simulink model "VehCtrl20260630_18B"  (R2018b)
settings: Solver=FixedStepAuto  StartTime=0.0  StopTime=inf  FixedStep=0.005  RelTol=1e-3
InitFcn:
  | mbd_mpc_consistency_checks(bdroot(gcs));
undefined symbols (not defined in the file): ANG_DEAD, BMS_NormalPwr, BrakeDeadZone, BrkPrsByBrkPct_TB_X, BrkPrsByBrkPct_TB_Y, DELAY_DISCHARGE, DELAY_RCUOFF, DRV_BACKWARD, DRV_BRAKE, DRV_FORWARD, DRV_NEUTRAL, DRV_PARK, DRV_UNPARK, DRV_ZEROTURN, EPB_LOCK, EPB_UNLOCK, ExtraLoadPwr, FanOff, fifo_0_vect, fifo_1_vect, HiFanReq, HV_finished, HV_No_Active, HV_POWER_OFF, HV_POWER_ON, HVDown, HVON, KaTLS_v_DrgUp_X_VehSpd, KeFTM_s_Way1OffDlyTime, KeFTM_TK_Way1CoolLv2OffBatTemp, KeFTM_TK_Way1CoolLv2OffMtrTemp, KeFTM_TK_Way1CoolLv2OnBatTemp, KeFTM_TK_Way1CoolLv2OnMtrTemp, KeFTM_TK_Way1CoolLv3OffBatTemp, KeFTM_TK_Way1CoolLv3OffMtrTemp, KeFTM_TK_Way1CoolLv3OnBatTemp, KeFTM_TK_Way1CoolLv3OnMtrTemp, KeFTM_TK_Way1CoolLv4OffBatTemp, KeFTM_TK_Way1CoolLv4OffMtrTemp, KeFTM_TK_Way1CoolLv4OnBatTemp, KeFTM_TK_Way1CoolLv4OnMtrTemp, Kp1, Kp2, LowFanReq, LQFP, MtrCmdGainFL, MtrCmdGainFR, MtrCmdGainRL, MtrCmdGainRR, MtrPwrFactor_RCU, MtrPwrHighToMidThd, MtrPwrLowToMidThd, MtrPwrMidToHighThd, MtrPwrMidToLowThd, MtrTrqMax, PCT_DEAD, Precharge, PTO_1000, PTO_540, pts1_fifo_0_vect ... (+32)
libraries: mbd_mpc574x_ec_toolbox x175, simulink x110, canmsglib x70
(part 8 of 15)

== system VehCtrl20260630_18B/SigIn/CAN0/DC-DC_Msg/UNPACK ==
  ID : Inport
  data : Inport  Port=2
  length : Inport  Port=3
  timestamp : Inport  Port=4
  Action Port : ActionPort  ActionType=case
  Add : Sum
  Bus Creator : BusCreator  Inputs=7  OutDataTypeStr=Bus: CAN_MESSAGE_BUS  NonVirtualBus=on
  Bus Creator1 : BusCreator  Inputs=8
  CAN Unpack6 : canmsglib/CAN Unpack  CANdbFile=E:\硕士工作\0.本周工作\20260428_changchun\VCU_260508_ChangChun\CAN协议0509\DCDC\DCDC_DBC_VCU_CAN0.dbc  MsgList=DCDC_msg1  MsgName=DCDC_msg1  MsgIDType=Extended (29-bit identifier)  MsgIdentifier=418931243  MsgLength=8  SignalInfo=DCDC_BasicSts$5$3$1$2$1$0$1$0$0$7$#DCDC_ErrorLevel$3$2$1$2$1$0$1$0$0$3$#DCDC_FaultLevel$48$8$1$2$1$0$1$0$0$200$#DCDC_Mdltem$8$8$1$2$1$0$1$-40$-40$150$#DCDC_Optcur$32$16$1$2$1$0$5.000000e-02$0$0$3.276750e+03$#DCDC_Optvol$16$16$1$2$1$0$5.000000e-02$0$0$3.276750e+03$#DCDC_Sfwver$56$8$1$2$1$0$1$0$1$255$#DCDC_WrkSts$1$2$1$2$1$0$1$0$0$3$#Spare$0$1$1$2$1$0$1$0$0$1$#  NSignals=9  IDPort=off  TimestampPort=off  ErrorPort=off  RemotePort=off  LengthPort=off  StatusPort=off  StartBits=str2num('[int32(5);int32(3);int32(48);int32(8);int32(32);int32(16);int32(56);int32(1);int32(0)]')  SignalSizes=str2num('[int32(3);int32(2);int32(8);int32(8);int32(16);int32(16);int32(8);int32(2);int32(1)]')  ByteOrders=str2num('[int32(1);int32(1);int32(1);int32(1);int32(1);int32(1);int32(1);int32(1);int32(1)]')  DataTypes=str2num('[int32(2);int32(2);int32(2);int32(2);int32(2);int32(2);int32(2);int32(2);int32(2)]')  MultiplexTypes=str2num('[int32(1);int32(1);int32(1);int32(1);int32(1);int32(1);int32(1);int32(1);int32(1)]')  MultiplexValues=str2num('[double(0);double(0);double(0);double(0);double(0);double(0);double(0);double(0);double(0)]')  Factors=str2num('[double(1);double(1);double(1);double(1);double(5.000000e-02);double(5.000000e-02);double(1);double(1);double(1)]')  Offsets=str2num('[double(0);double(0);double(0);double(-40);double(0);double(0);double(0);double(0);double(0)]')  Minimums=str2num('[double(0);double(0);double(0);double(-40);double(0);double(0);double(1);double(0);double(0)]')  Maximums=str2num('[double(7);double(3);double(200);double(150);double(3.276750e+03);double(3.276750e+03);double(255);double(3);double(1)]')  ApplyMinMax=off
      settings: SourceProductName=Simulink Real-Time  SourceProductBaseCode=XP  DataFormat=CANdb specified signals
  Constant : Constant  OutDataTypeStr=uint8
  Constant1 : Constant  OutDataTypeStr=uint8
  Constant4 : Constant  Value=0  OutDataTypeStr=uint8
  Constant5 : Constant  Value=0  OutDataTypeStr=uint8
  Data Store Read : DataStoreRead  DataStoreName=Cnt_DCDC
  Data Store Write : DataStoreWrite  DataStoreName=Cnt_DCDC
  Data Type Conversion{,14..15,17} (4 alike) : DataTypeConversion  OutDataTypeStr=uint8
  Data Type Conversion{1..6,61..62} (8 alike) : DataTypeConversion  OutDataTypeStr=single
  Data Type Conversion18 : DataTypeConversion  OutDataTypeStr=uint32
  Data Type Conversion19 : DataTypeConversion  OutDataTypeStr=double
  Terminator : Terminator
  Message : Outport
  wires:
  Constant4/1 -> Data Type Conversion15/1
  length/1 -> Data Type Conversion14/1
  data/1 -> Bus Creator/7  "Data"
  Data Type Conversion18/1 -> Bus Creator/5  "ID"
  Constant1/1 -> Data Type Conversion/1
  Constant5/1 -> Data Type Conversion17/1
  ID/1 -> Data Type Conversion18/1
  Data Type Conversion19/1 -> Bus Creator/6  "Timestamp"
  timestamp/1 -> Data Type Conversion19/1
  Data Type Conversion17/1 -> Bus Creator/4  "Error"
  Bus Creator/1 -> CAN Unpack6/1  "CAN_Msg_In"
  Data Type Conversion/1 -> Bus Creator/1  "Extended"
  Data Type Conversion14/1 -> Bus Creator/2  "Length"
  Data Type Conversion15/1 -> Bus Creator/3  "Remote"
  Bus Creator1/1 -> Message/1
  Data Type Conversion4/1 -> Bus Creator1/1  "DCDC_BasicSts"
  Data Type Conversion61/1 -> Bus Creator1/2  "DCDC_ErrorLevel"
  Data Type Conversion62/1 -> Bus Creator1/3  "DCDC_FaultLevel"
  Data Type Conversion2/1 -> Bus Creator1/4  "DCDC_Mdltem"
  Data Type Conversion1/1 -> Bus Creator1/5  "DCDC_Optcur"
  CAN Unpack6/9 -> Terminator/1
  Data Type Conversion3/1 -> Bus Creator1/6  "DCDC_Optvol"
  Data Type Conversion5/1 -> Bus Creator1/7  "DCDC_Sfwver"
  Data Type Conversion6/1 -> Bus Creator1/8  "DCDC_WrkSts"
  CAN Unpack6/1 -> Data Type Conversion4/1
  CAN Unpack6/2 -> Data Type Conversion61/1
  CAN Unpack6/3 -> Data Type Conversion62/1
  CAN Unpack6/4 -> Data Type Conversion2/1
  CAN Unpack6/5 -> Data Type Conversion1/1
  CAN Unpack6/6 -> Data Type Conversion3/1
  CAN Unpack6/7 -> Data Type Conversion5/1
  CAN Unpack6/8 -> Data Type Conversion6/1
  Add/1 -> Data Store Write/1
  Constant/1 -> Add/2
  Data Store Read/1 -> Add/1

== system VehCtrl20260630_18B/SigIn/CAN0/PTC1/UNPACK ==
  ID : Inport
  data : Inport  Port=2
  length : Inport  Port=3
  timestamp : Inport  Port=4
  Action Port : ActionPort  ActionType=case
  Bus Creator : BusCreator  Inputs=7  OutDataTypeStr=Bus: CAN_MESSAGE_BUS  NonVirtualBus=on
  Bus Creator1 : BusCreator  Inputs=7
  CAN Unpack6 : canmsglib/CAN Unpack  CANdbFile=D:\VCU\VCU_AgriculturalMachinery_ChangChun\CAN协议8.4\PTC\PTC_Sheet1.dbc  MsgList=PTC_1  MsgName=PTC_1  MsgIDType=Standard (11-bit identifier)  MsgIdentifier=1179  MsgLength=8  SignalInfo=PTC_Actualdutycycle$56$8$2$2$1$0$1$0$0$100$#PTC_Consumedpower$24$16$2$2$1$0$2$0$0$16000$#PTC_Coolanttemperature$48$8$2$2$1$0$1$-40$0$140$#PTC_IGBTheatsinktemperature$40$8$2$2$1$0$1$-40$0$140$#PTC_Operatingcurrent$0$8$2$2$1$0$2.000000e-01$0$0$50$#PTC_Workingcurrent$8$8$2$2$1$0$2.000000e-01$0$0$50$#PTC_Workingvoltage$16$8$2$2$1$0$4$0$0$1000$#  NSignals=7  IDPort=off  TimestampPort=off  ErrorPort=off  RemotePort=off  LengthPort=off  StatusPort=off  StartBits=str2num('[int32(56);int32(24);int32(48);int32(40);int32(0);int32(8);int32(16)]')  SignalSizes=str2num('[int32(8);int32(16);int32(8);int32(8);int32(8);int32(8);int32(8)]')  ByteOrders=str2num('[int32(2);int32(2);int32(2);int32(2);int32(2);int32(2);int32(2)]')  DataTypes=str2num('[int32(2);int32(2);int32(2);int32(2);int32(2);int32(2);int32(2)]')  MultiplexTypes=str2num('[int32(1);int32(1);int32(1);int32(1);int32(1);int32(1);int32(1)]')  MultiplexValues=str2num('[double(0);double(0);double(0);double(0);double(0);double(0);double(0)]')  Factors=str2num('[double(1);double(2);double(1);double(1);double(2.000000e-01);double(2.000000e-01);double(4)]')  Offsets=str2num('[double(0);double(0);double(-40);double(-40);double(0);double(0);double(0)]')  Minimums=str2num('[double(0);double(0);double(0);double(0);double(0);double(0);double(0)]')  Maximums=str2num('[double(100);double(16000);double(140);double(140);double(50);double(50);double(1000)]')  ApplyMinMax=off
      settings: SourceProductName=Simulink Real-Time  SourceProductBaseCode=XP  DataFormat=CANdb specified signals
  Constant1 : Constant  OutDataTypeStr=uint8
  Constant4 : Constant  Value=0  OutDataTypeStr=uint8
  Constant5 : Constant  Value=0  OutDataTypeStr=uint8
  Data Type Conversion{,14..15,17} (4 alike) : DataTypeConversion  OutDataTypeStr=uint8
  Data Type Conversion{1..5,61..62} (7 alike) : DataTypeConversion  OutDataTypeStr=single
  Data Type Conversion18 : DataTypeConversion  OutDataTypeStr=uint32
  Data Type Conversion19 : DataTypeConversion  OutDataTypeStr=double
  Message : Outport
  wires:
  Constant4/1 -> Data Type Conversion15/1
  length/1 -> Data Type Conversion14/1
  data/1 -> Bus Creator/7  "Data"
  Data Type Conversion18/1 -> Bus Creator/5  "ID"
  Constant1/1 -> Data Type Conversion/1
  Constant5/1 -> Data Type Conversion17/1
  ID/1 -> Data Type Conversion18/1
  Data Type Conversion19/1 -> Bus Creator/6  "Timestamp"
  timestamp/1 -> Data Type Conversion19/1
  Data Type Conversion17/1 -> Bus Creator/4  "Error"
  Bus Creator/1 -> CAN Unpack6/1  "CAN_Msg_In"
  Data Type Conversion/1 -> Bus Creator/1  "Extended"
  Data Type Conversion14/1 -> Bus Creator/2  "Length"
  Data Type Conversion15/1 -> Bus Creator/3  "Remote"
  Bus Creator1/1 -> Message/1
  Data Type Conversion4/1 -> Bus Creator1/1  "PTC_Actualdutycycle"
  Data Type Conversion61/1 -> Bus Creator1/2  "PTC_Consumedpower"
  Data Type Conversion62/1 -> Bus Creator1/3  "PTC_Coolanttemperature"
  Data Type Conversion2/1 -> Bus Creator1/4  "PTC_IGBTheatsinktemperature"
  Data Type Conversion1/1 -> Bus Creator1/5  "PTC_Operatingcurrent"
  Data Type Conversion3/1 -> Bus Creator1/6  "PTC_Workingcurrent"
  Data Type Conversion5/1 -> Bus Creator1/7  "PTC_Workingvoltage"
  CAN Unpack6/1 -> Data Type Conversion4/1
  CAN Unpack6/2 -> Data Type Conversion61/1
  CAN Unpack6/3 -> Data Type Conversion62/1
  CAN Unpack6/4 -> Data Type Conversion2/1
  CAN Unpack6/5 -> Data Type Conversion1/1
  CAN Unpack6/6 -> Data Type Conversion3/1
  CAN Unpack6/7 -> Data Type Conversion5/1

== system VehCtrl20260630_18B/SigIn/CAN0/PTC2/UNPACK ==
  ID : Inport
  data : Inport  Port=2
  length : Inport  Port=3
  timestamp : Inport  Port=4
  Action Port : ActionPort  ActionType=case
  Bus Creator : BusCreator  Inputs=7  OutDataTypeStr=Bus: CAN_MESSAGE_BUS  NonVirtualBus=on
  Bus Creator1 : BusCreator  Inputs=11
  CAN Unpack6 : canmsglib/CAN Unpack  CANdbFile=D:\VCU\VCU_AgriculturalMachinery_ChangChun\CAN协议8.4\PTC\PTC_Sheet1.dbc  MsgList=PTC_2  MsgName=PTC_2  MsgIDType=Standard (11-bit identifier)  MsgIdentifier=1180  MsgLength=4  SignalInfo=PTC_Highvoltagecircuitdisconnection$6$2$2$2$1$0$1$0$0$3$#PTC_Highvoltagepowersupplycondition$4$2$2$2$1$0$1$0$0$3$#PTC_IG1powersupplyisfaulty$14$2$2$2$1$0$1$0$0$3$#PTC_IGBTshortcircuit$18$1$2$2$1$0$1$0$0$1$#PTC_Numberofsoftwaremodifications$24$8$2$2$1$0$1$0$0$255$#PTC_Requesttodisconnecttheairconditionercontactor$16$2$2$2$1$0$1$0$0$3$#PTC_coolanttemperaturesensorisfaulty$12$2$2$2$1$0$1$0$0$3$#PTC_enabledSts$0$2$2$2$1$0$1$0$0$3$#PTC_faultySts$2$2$2$2$1$0$1$0$0$3$#TheIGBTtemperaturesensorisfaulty$10$2$2$2$1$0$1$0$0$3$#Thecommunicationwiththeairconditionercontrollerislost$8$2$2$2$1$0$1$0$0$3$#  NSignals=11  IDPort=off  TimestampPort=off  ErrorPort=off  RemotePort=off  LengthPort=off  StatusPort=off  StartBits=str2num('[int32(6);int32(4);int32(14);int32(18);int32(24);int32(16);int32(12);int32(0);int32(2);int32(10);int32(8)]')  SignalSizes=str2num('[int32(2);int32(2);int32(2);int32(1);int32(8);int32(2);int32(2);int32(2);int32(2);int32(2);int32(2)]')  ByteOrders=str2num('[int32(2);int32(2);int32(2);int32(2);int32(2);int32(2);int32(2);int32(2);int32(2);int32(2);int32(2)]')  DataTypes=str2num('[int32(2);int32(2);int32(2);int32(2);int32(2);int32(2);int32(2);int32(2);int32(2);int32(2);int32(2)]')  MultiplexTypes=str2num('[int32(1);int32(1);int32(1);int32(1);int32(1);int32(1);int32(1);int32(1);int32(1);int32(1);int32(1)]')  MultiplexValues=str2num('[double(0);double(0);double(0);double(0);double(0);double(0);double(0);double(0);double(0);double(0);double(0)]')  Factors=str2num('[double(1);double(1);double(1);double(1);double(1);double(1);double(1);double(1);double(1);double(1);double(1)]')  Offsets=str2num('[double(0);double(0);double(0);double(0);double(0);double(0);double(0);double(0);double(0);double(0);double(0)]')  Minimums=str2num('[double(0);double(0);double(0);double(0);double(0);double(0);double(0);double(0);double(0);double(0);double(0)]')  Maximums=str2num('[double(3);double(3);double(3);double(1);double(255);double(3);double(3);double(3);double(3);double(3);double(3)]')  ApplyMinMax=off
      settings: SourceProductName=Simulink Real-Time  SourceProductBaseCode=XP  DataFormat=CANdb specified signals
  Constant1 : Constant  OutDataTypeStr=uint8
  Constant4 : Constant  Value=0  OutDataTypeStr=uint8
  Constant5 : Constant  Value=0  OutDataTypeStr=uint8
  Data Type Conversion{,2..9,14..15,17,61..62} (14 alike) : DataTypeConversion  OutDataTypeStr=uint8
  Data Type Conversion1 : DataTypeConversion  OutDataTypeStr=single
  Data Type Conversion18 : DataTypeConversion  OutDataTypeStr=uint32
  Data Type Conversion19 : DataTypeConversion  OutDataTypeStr=double
  Message : Outport
  wires:
  Constant4/1 -> Data Type Conversion15/1
  length/1 -> Data Type Conversion14/1
  data/1 -> Bus Creator/7  "Data"
  Data Type Conversion18/1 -> Bus Creator/5  "ID"
  Constant1/1 -> Data Type Conversion/1
  Constant5/1 -> Data Type Conversion17/1
  ID/1 -> Data Type Conversion18/1
  Data Type Conversion19/1 -> Bus Creator/6  "Timestamp"
  timestamp/1 -> Data Type Conversion19/1
  Data Type Conversion17/1 -> Bus Creator/4  "Error"
  Bus Creator/1 -> CAN Unpack6/1  "CAN_Msg_In"
  Data Type Conversion/1 -> Bus Creator/1  "Extended"
  Data Type Conversion14/1 -> Bus Creator/2  "Length"
  Data Type Conversion15/1 -> Bus Creator/3  "Remote"
  Bus Creator1/1 -> Message/1
  Data Type Conversion4/1 -> Bus Creator1/1  "PTC_Highvoltagepowersupplycondition"
  Data Type Conversion61/1 -> Bus Creator1/2  "PTC_Highvoltagecircuitdisconnection"
  Data Type Conversion62/1 -> Bus Creator1/3  "PTC_IG1powersupplyisfaulty"
  Data Type Conversion2/1 -> Bus Creator1/4  "PTC_IGBTshortcircuit"
  Data Type Conversion1/1 -> Bus Creator1/5  "PTC_Numberofsoftwaremodifications"
  CAN Unpack6/9 -> Data Type Conversion7/1
  Data Type Conversion3/1 -> Bus Creator1/6  "PTC_Requesttodisconnecttheairconditionercontactor"
  Data Type Conversion5/1 -> Bus Creator1/7  "PTC_coolanttemperaturesensorisfaulty"
  Data Type Conversion6/1 -> Bus Creator1/8  "PTC_enabledSts"
  CAN Unpack6/1 -> Data Type Conversion4/1
  CAN Unpack6/2 -> Data Type Conversion61/1
  CAN Unpack6/3 -> Data Type Conversion62/1
  CAN Unpack6/4 -> Data Type Conversion2/1
  CAN Unpack6/5 -> Data Type Conversion1/1
  CAN Unpack6/6 -> Data Type Conversion3/1
  CAN Unpack6/7 -> Data Type Conversion5/1
  CAN Unpack6/8 -> Data Type Conversion6/1
  Data Type Conversion7/1 -> Bus Creator1/9  "PTC_faulty Sts"
  Data Type Conversion8/1 -> Bus Creator1/10  "TheIGBTtemperaturesensorisfaulty"
  CAN Unpack6/10 -> Data Type Conversion8/1
  Data Type Conversion9/1 -> Bus Creator1/11  "Thecommunicationwiththeairconditionercontrollerislost"
  CAN Unpack6/11 -> Data Type Conversion9/1

== system VehCtrl20260630_18B/SigIn/CAN0/RMT_VCU1/UNPACK ==
  ID : Inport
  data : Inport  Port=2
  length : Inport  Port=3
  timestamp : Inport  Port=4
  Action Port : ActionPort  ActionType=case
  Add : Sum
  Bus Creator : BusCreator  Inputs=7  OutDataTypeStr=Bus: CAN_MESSAGE_BUS  NonVirtualBus=on
  Bus Creator1 : BusCreator  Inputs=3
  CAN Unpack6 : canmsglib/CAN Unpack  CANdbFile=E:\硕士工作\0.本周工作\20260428_changchun\VCU_260508_ChangChun\CAN协议0430\RMT\CAN_Matrix_Sheet1_0509.dbc  MsgList=JoyStick  MsgName=JoyStick  MsgIDType=Standard (11-bit identifier)  MsgIdentifier=1  MsgLength=8  SignalInfo=CmdAccBrkPct$32$16$1$2$1$0$1$0$0$100$#CmdSteerAng$0$16$1$2$1$0$1$0$0$100$#ReserveL$48$16$1$2$1$0$1$0$0$100$#ReserveR$16$16$1$2$1$0$1$0$0$100$#  NSignals=4  IDPort=off  TimestampPort=off  ErrorPort=off  RemotePort=off  LengthPort=off  StatusPort=off  StartBits=str2num('[int32(32);int32(0);int32(48);int32(16)]')  SignalSizes=str2num('[int32(16);int32(16);int32(16);int32(16)]')  ByteOrders=str2num('[int32(1);int32(1);int32(1);int32(1)]')  DataTypes=str2num('[int32(2);int32(2);int32(2);int32(2)]')  MultiplexTypes=str2num('[int32(1);int32(1);int32(1);int32(1)]')  MultiplexValues=str2num('[double(0);double(0);double(0);double(0)]')  Factors=str2num('[double(1);double(1);double(1);double(1)]')  Offsets=str2num('[double(0);double(0);double(0);double(0)]')  Minimums=str2num('[double(0);double(0);double(0);double(0)]')  Maximums=str2num('[double(100);double(100);double(100);double(100)]')  ApplyMinMax=off
      settings: SourceProductName=Simulink Real-Time  SourceProductBaseCode=XP  DataFormat=CANdb specified signals
  Constant : Constant  OutDataTypeStr=uint8
  Constant1 : Constant  Value=0  OutDataTypeStr=uint8
  Constant4 : Constant  Value=0  OutDataTypeStr=uint8
  Constant5 : Constant  Value=0  OutDataTypeStr=uint8
  Data Store Read : DataStoreRead  DataStoreName=Cnt_RMT1
  Data Store Write : DataStoreWrite  DataStoreName=Cnt_RMT1
  Data Type Conversion{,14..15,17} (4 alike) : DataTypeConversion  OutDataTypeStr=uint8
  Data Type Conversion1 : DataTypeConversion  OutDataTypeStr=single
  Data Type Conversion18 : DataTypeConversion  OutDataTypeStr=uint32
  Data Type Conversion19 : DataTypeConversion  OutDataTypeStr=double
  Data Type Conversion61 : DataTypeConversion  OutDataTypeStr=single
  Subsystem : Subsystem
  Subsystem1 : Subsystem
  Subsystem2 : Subsystem
  Terminator : Terminator
  Terminator1 : Terminator
  Message : Outport
  wires:
  Constant4/1 -> Data Type Conversion15/1
  length/1 -> Data Type Conversion14/1
  data/1 -> Bus Creator/7  "Data"
  Data Type Conversion18/1 -> Bus Creator/5  "ID"
  Constant1/1 -> Data Type Conversion/1
  Constant5/1 -> Data Type Conversion17/1
  ID/1 -> Data Type Conversion18/1
  Data Type Conversion19/1 -> Bus Creator/6  "Timestamp"
  timestamp/1 -> Data Type Conversion19/1
  Data Type Conversion17/1 -> Bus Creator/4  "Error"
  Bus Creator/1 -> CAN Unpack6/1  "CAN_Msg_In"
  Data Type Conversion/1 -> Bus Creator/1  "Extended"
  Data Type Conversion14/1 -> Bus Creator/2  "Length"
  Data Type Conversion15/1 -> Bus Creator/3  "Remote"
  Bus Creator1/1 -> Message/1
  Data Type Conversion61/1 -> Subsystem1/1(In1), Subsystem/1(In1)  "RMT_CmdAccBrkSig"
  Subsystem2/1(Out1) -> Bus Creator1/3  "RMT_CmdStrAng"
  CAN Unpack6/1 -> Data Type Conversion61/1
  Add/1 -> Data Store Write/1
  Constant/1 -> Add/2
  Data Store Read/1 -> Add/1
  Subsystem/1(Out1) -> Bus Creator1/1  "RMT_CmdAccPct"
  Subsystem1/1(Out1) -> Bus Creator1/2  "RMT_CmdBrkPct"
  CAN Unpack6/2 -> Data Type Conversion1/1
  Data Type Conversion1/1 -> Subsystem2/1(In1)  "RMT_CmdStrSig"
  CAN Unpack6/3 -> Terminator/1
  CAN Unpack6/4 -> Terminator1/1

== system VehCtrl20260630_18B/SigIn/CAN0/RMT_VCU2/UNPACK ==
  ID : Inport
  data : Inport  Port=2
  length : Inport  Port=3
  timestamp : Inport  Port=4
  Action Port : ActionPort  ActionType=case
  Add : Sum
  Bus Creator : BusCreator  Inputs=7  OutDataTypeStr=Bus: CAN_MESSAGE_BUS  NonVirtualBus=on
  Bus Creator1 : BusCreator  Inputs=3
  CAN Unpack6 : canmsglib/CAN Unpack  CANdbFile=E:\硕士工作\0.本周工作\20260428_changchun\VCU_260508_ChangChun\CAN协议0430\RMT\CAN_Matrix_Sheet1_0509.dbc  MsgList=VR  MsgName=VR  MsgIDType=Standard (11-bit identifier)  MsgIdentifier=2  MsgLength=8  SignalInfo=CmdLiftPct$32$16$1$2$1$0$1$0$0$100$#CmdTrackWidthPct$0$16$1$2$1$0$1$0$0$100$#MotorTorqueGear$16$16$1$2$1$0$1$0$0$100$#ReserveVRB$48$16$1$2$1$0$1$0$0$100$#  NSignals=4  IDPort=off  TimestampPort=off  ErrorPort=off  RemotePort=off  LengthPort=off  StatusPort=off  StartBits=str2num('[int32(32);int32(0);int32(16);int32(48)]')  SignalSizes=str2num('[int32(16);int32(16);int32(16);int32(16)]')  ByteOrders=str2num('[int32(1);int32(1);int32(1);int32(1)]')  DataTypes=str2num('[int32(2);int32(2);int32(2);int32(2)]')  MultiplexTypes=str2num('[int32(1);int32(1);int32(1);int32(1)]')  MultiplexValues=str2num('[double(0);double(0);double(0);double(0)]')  Factors=str2num('[double(1);double(1);double(1);double(1)]')  Offsets=str2num('[double(0);double(0);double(0);double(0)]')  Minimums=str2num('[double(0);double(0);double(0);double(0)]')  Maximums=str2num('[double(100);double(100);double(100);double(100)]')  ApplyMinMax=off
      settings: SourceProductName=Simulink Real-Time  SourceProductBaseCode=XP  DataFormat=CANdb specified signals
  Constant : Constant  OutDataTypeStr=uint8
  Constant1 : Constant  Value=0  OutDataTypeStr=uint8
  Constant4 : Constant  Value=0  OutDataTypeStr=uint8
  Constant5 : Constant  Value=0  OutDataTypeStr=uint8
  Data Store Read : DataStoreRead  DataStoreName=Cnt_RMT2
  Data Store Write : DataStoreWrite  DataStoreName=Cnt_RMT2
  Data Store Write1 : DataStoreWrite  Commented=on  DataStoreName=MtrTrqGr
  Data Type Conversion{,14..15,17} (4 alike) : DataTypeConversion  OutDataTypeStr=uint8
  Data Type Conversion1 : DataTypeConversion  OutDataTypeStr=single
  Data Type Conversion18 : DataTypeConversion  OutDataTypeStr=uint32
  Data Type Conversion19 : DataTypeConversion  OutDataTypeStr=double
  Data Type Conversion2 : DataTypeConversion  OutDataTypeStr=single
  Data Type Conversion3 : DataTypeConversion  OutDataTypeStr=single
  Subsystem : Subsystem
  Subsystem3 : Subsystem
  Subsystem4 : Subsystem
  Terminator : Terminator
  Message : Outport
  wires:
  Bus Creator1/1 -> Message/1
  Data Type Conversion15/1 -> Bus Creator/3  "Remote"
  Data Type Conversion14/1 -> Bus Creator/2  "Length"
  Data Type Conversion/1 -> Bus Creator/1  "Extended"
  Bus Creator/1 -> CAN Unpack6/1  "CAN_Msg_In"
  Data Type Conversion17/1 -> Bus Creator/4  "Error"
  timestamp/1 -> Data Type Conversion19/1
  Data Type Conversion19/1 -> Bus Creator/6  "Timestamp"
  ID/1 -> Data Type Conversion18/1
  Constant5/1 -> Data Type Conversion17/1
  Constant1/1 -> Data Type Conversion/1
  Data Type Conversion18/1 -> Bus Creator/5  "ID"
  data/1 -> Bus Creator/7  "Data"
  length/1 -> Data Type Conversion14/1
  Constant4/1 -> Data Type Conversion15/1
  Add/1 -> Data Store Write/1
  Constant/1 -> Add/2
  Data Store Read/1 -> Add/1
  Data Type Conversion1/1 -> Subsystem/1(RMT_MtrTqGr)
  Subsystem/1(Out1) -> Data Store Write1/1, Bus Creator1/3  "RMT_MtrTqGr"
  CAN Unpack6/4 -> Terminator/1
  CAN Unpack6/3 -> Data Type Conversion1/1
  Data Type Conversion3/1 -> Subsystem3/1(In1)  "RMT_CmdLiftSig"
  Subsystem3/1(Out1) -> Bus Creator1/1  "RMT_ModeSusp"
  CAN Unpack6/1 -> Data Type Conversion3/1
  Subsystem4/1(Out1) -> Bus Creator1/2  "RMT_ModeWidth"
  Data Type Conversion2/1 -> Subsystem4/1(In1)  "RMT_CmdWidthSig"
  CAN Unpack6/2 -> Data Type Conversion2/1

== system VehCtrl20260630_18B/SigIn/CAN0/RMT_VCU3/UNPACK ==
  note: 1 - 自动驾驶
      | 0 - 遥控
  note: 1 - 急停
      | 0 - 无效
  ID : Inport
  data : Inport  Port=2
  length : Inport  Port=3
  timestamp : Inport  Port=4
  Action Port : ActionPort  ActionType=case
  Add : Sum
  Bus Creator : BusCreator  Inputs=7  OutDataTypeStr=Bus: CAN_MESSAGE_BUS  NonVirtualBus=on
  Bus Creator1 : BusCreator  Inputs=4
  CAN Unpack6 : canmsglib/CAN Unpack  CANdbFile=D:\VCU\VCU_AgriculturalMachinery_ChangChun\VCU_AgriculturalMachinery_260520_ChangChun\CAN协议0520\RMT\RMT_dbc1.dbc  MsgList=SW1  MsgName=SW1  MsgIDType=Standard (11-bit identifier)  MsgIdentifier=3  MsgLength=8  SignalInfo=CoachSwitch$48$16$1$2$1$0$1$0$0$100$#EmStop$16$16$1$2$1$0$1$0$0$100$#ModeDirection$0$16$1$2$1$0$1$0$0$100$#ReserveH$32$16$1$2$1$0$1$0$0$100$#  NSignals=4  IDPort=off  TimestampPort=off  ErrorPort=off  RemotePort=off  LengthPort=off  StatusPort=off  StartBits=str2num('[int32(48);int32(16);int32(0);int32(32)]')  SignalSizes=str2num('[int32(16);int32(16);int32(16);int32(16)]')  ByteOrders=str2num('[int32(1);int32(1);int32(1);int32(1)]')  DataTypes=str2num('[int32(2);int32(2);int32(2);int32(2)]')  MultiplexTypes=str2num('[int32(1);int32(1);int32(1);int32(1)]')  MultiplexValues=str2num('[double(0);double(0);double(0);double(0)]')  Factors=str2num('[double(1);double(1);double(1);double(1)]')  Offsets=str2num('[double(0);double(0);double(0);double(0)]')  Minimums=str2num('[double(0);double(0);double(0);double(0)]')  Maximums=str2num('[double(100);double(100);double(100);double(100)]')  ApplyMinMax=off
      settings: SourceProductName=Simulink Real-Time  SourceProductBaseCode=XP  DataFormat=CANdb specified signals
  Constant : Constant  OutDataTypeStr=uint8
  Constant1 : Constant  Value=0  OutDataTypeStr=uint8
  Constant4 : Constant  Value=0  OutDataTypeStr=uint8
  Constant5 : Constant  Value=0  OutDataTypeStr=uint8
  Data Store Read : DataStoreRead  DataStoreName=Cnt_RMT3
  Data Store Write : DataStoreWrite  DataStoreName=Cnt_RMT3
  Data Store Write1 : DataStoreWrite  DataStoreName=EmStop_RMT
  Data Type Conversion{,14..15,17} (4 alike) : DataTypeConversion  OutDataTypeStr=uint8
  Data Type Conversion{1,3,6..7} (4 alike) : DataTypeConversion  OutDataTypeStr=single
  Data Type Conversion18 : DataTypeConversion  OutDataTypeStr=uint32
  Data Type Conversion19 : DataTypeConversion  OutDataTypeStr=double
  Subsystem1 : Subsystem
  Subsystem2 : Subsystem
  Subsystem4 : Subsystem
  Subsystem5 : Subsystem
  Message : Outport
  wires:
  Constant4/1 -> Data Type Conversion15/1
  length/1 -> Data Type Conversion14/1
  data/1 -> Bus Creator/7  "Data"
  Data Type Conversion18/1 -> Bus Creator/5  "ID"
  Constant1/1 -> Data Type Conversion/1
  Constant5/1 -> Data Type Conversion17/1
  ID/1 -> Data Type Conversion18/1
  Data Type Conversion19/1 -> Bus Creator/6  "Timestamp"
  timestamp/1 -> Data Type Conversion19/1
  Data Type Conversion17/1 -> Bus Creator/4  "Error"
  Bus Creator/1 -> CAN Unpack6/1  "CAN_Msg_In"
  Data Type Conversion/1 -> Bus Creator/1  "Extended"
  Data Type Conversion14/1 -> Bus Creator/2  "Length"
  Data Type Conversion15/1 -> Bus Creator/3  "Remote"
  Add/1 -> Data Store Write/1
  Constant/1 -> Add/2
  Data Store Read/1 -> Add/1
  Data Type Conversion3/1 -> Subsystem1/1(In1)  "RMT_G"
  Bus Creator1/1 -> Message/1
  Data Type Conversion6/1 -> Subsystem4/1(In1)  "RMT_B"
  Data Type Conversion7/1 -> Subsystem5/1(In1)  "RMT_A"
  Subsystem2/1(Out1) -> Bus Creator1/1  "RMT_Auto"
  CAN Unpack6/1 -> Data Type Conversion1/1
  Data Type Conversion1/1 -> Subsystem2/1(In1)  "RMT_H"
  CAN Unpack6/3 -> Data Type Conversion6/1
  Subsystem4/1(Out1) -> Bus Creator1/3  "RMT_ModeDirection"
  Subsystem5/1(Out1) -> Data Store Write1/1, Bus Creator1/2  "RMT_EmStop"
  Subsystem1/1(Out1) -> Bus Creator1/4  "ReserveH"
  CAN Unpack6/4 -> Data Type Conversion3/1
  CAN Unpack6/2 -> Data Type Conversion7/1

== system VehCtrl20260630_18B/SigIn/CAN0/RMT_VCU4/UNPACK ==
  ID : Inport
  data : Inport  Port=2
  length : Inport  Port=3
  timestamp : Inport  Port=4
  Action Port : ActionPort  ActionType=case
  Add : Sum
  Bus Creator : BusCreator  Inputs=7  OutDataTypeStr=Bus: CAN_MESSAGE_BUS  NonVirtualBus=on
  Bus Creator1 : BusCreator  Inputs=3
  CAN Unpack6 : canmsglib/CAN Unpack  CANdbFile=D:\VCU\VCU_AgriculturalMachinery_ChangChun\VCU_AgriculturalMachinery_260520_ChangChun\CAN协议0520\RMT\RMT_dbc1.dbc  MsgList=SW2  MsgName=SW2  MsgIDType=Standard (11-bit identifier)  MsgIdentifier=4  MsgLength=8  SignalInfo=ModeSafety$0$16$1$2$1$0$1$0$0$100$#PowerSwitch$32$16$1$2$1$0$1$0$0$100$#PtoMode$16$16$1$2$1$0$1$0$0$100$#RangeExtenderMode$48$16$1$2$1$0$1$0$0$100$#  NSignals=4  IDPort=off  TimestampPort=off  ErrorPort=off  RemotePort=off  LengthPort=off  StatusPort=off  StartBits=str2num('[int32(0);int32(32);int32(16);int32(48)]')  SignalSizes=str2num('[int32(16);int32(16);int32(16);int32(16)]')  ByteOrders=str2num('[int32(1);int32(1);int32(1);int32(1)]')  DataTypes=str2num('[int32(2);int32(2);int32(2);int32(2)]')  MultiplexTypes=str2num('[int32(1);int32(1);int32(1);int32(1)]')  MultiplexValues=str2num('[double(0);double(0);double(0);double(0)]')  Factors=str2num('[double(1);double(1);double(1);double(1)]')  Offsets=str2num('[double(0);double(0);double(0);double(0)]')  Minimums=str2num('[double(0);double(0);double(0);double(0)]')  Maximums=str2num('[double(100);double(100);double(100);double(100)]')  ApplyMinMax=off
      settings: SourceProductName=Simulink Real-Time  SourceProductBaseCode=XP  DataFormat=CANdb specified signals
  Constant : Constant  OutDataTypeStr=uint8
  Constant1 : Constant  Value=0  OutDataTypeStr=uint8
  Constant4 : Constant  Value=0  OutDataTypeStr=uint8
  Constant5 : Constant  Value=0  OutDataTypeStr=uint8
  Data Store Read : DataStoreRead  DataStoreName=Cnt_RMT4
  Data Store Write : DataStoreWrite  DataStoreName=Cnt_RMT4
  Data Store Write1 : DataStoreWrite  DataStoreName=KeySW
  Data Type Conversion{,14..15,17} (4 alike) : DataTypeConversion  OutDataTypeStr=uint8
  Data Type Conversion{1,3..5} (4 alike) : DataTypeConversion  OutDataTypeStr=single
  Data Type Conversion18 : DataTypeConversion  OutDataTypeStr=uint32
  Data Type Conversion19 : DataTypeConversion  OutDataTypeStr=double
  Data Type Conversion2 : DataTypeConversion
  Subsystem1 : Subsystem
  Subsystem2 : Subsystem
  Subsystem3 : Subsystem
  Subsystem4 : Subsystem
  Message : Outport
  wires:
  Constant4/1 -> Data Type Conversion15/1
  length/1 -> Data Type Conversion14/1
  data/1 -> Bus Creator/7  "Data"
  Data Type Conversion18/1 -> Bus Creator/5  "ID"
  Constant1/1 -> Data Type Conversion/1
  Constant5/1 -> Data Type Conversion17/1
  ID/1 -> Data Type Conversion18/1
  Data Type Conversion19/1 -> Bus Creator/6  "Timestamp"
  timestamp/1 -> Data Type Conversion19/1
  Data Type Conversion17/1 -> Bus Creator/4  "Error"
  Bus Creator/1 -> CAN Unpack6/1  "CAN_Msg_In"
  Data Type Conversion/1 -> Bus Creator/1  "Extended"
  Data Type Conversion14/1 -> Bus Creator/2  "Length"
  Data Type Conversion15/1 -> Bus Creator/3  "Remote"
  Bus Creator1/1 -> Message/1
  Add/1 -> Data Store Write/1
  Constant/1 -> Add/2
  Data Store Read/1 -> Add/1
  Data Type Conversion1/1 -> Subsystem3/1(In1)  "RMT_A"
  Subsystem3/1(Out1) -> Data Type Conversion2/1
  Data Type Conversion2/1 -> Data Store Write1/1  "KeySW"
  Data Type Conversion5/1 -> Subsystem2/1(In1)
  Subsystem2/1(Out1) -> Bus Creator1/2  "RMT_PtoMode"
  Data Type Conversion3/1 -> Subsystem1/1(In1)
  Subsystem1/1(Out1) -> Bus Creator1/3  "RMT_RCU"
  Data Type Conversion4/1 -> Subsystem4/1(In1)
  Subsystem4/1(Out1) -> Bus Creator1/1  "ModeSafety"
  CAN Unpack6/2 -> Data Type Conversion1/1
  CAN Unpack6/3 -> Data Type Conversion5/1
  CAN Unpack6/4 -> Data Type Conversion3/1
  CAN Unpack6/1 -> Data Type Conversion4/1

== system VehCtrl20260630_18B/SigIn/CAN1/ACM_Msg/UNPACK ==
  ID : Inport
  data : Inport  Port=2
  length : Inport  Port=3
  timestamp : Inport  Port=4
  Action Port : ActionPort  ActionType=case
  Add : Sum
  Bus Creator : BusCreator  Inputs=7  OutDataTypeStr=Bus: CAN_MESSAGE_BUS  NonVirtualBus=on
  Bus Creator1 : BusCreator  Inputs=10
  CAN Unpack6 : canmsglib/CAN Unpack  CANdbFile=D:\VCU\VCU_AgriculturalMachinery_ChangChun\CAN协议8.4\空压机\ACM_CAN_1.0.dbc  MsgList=AC_0x284  MsgName=AC_0x284  MsgIDType=Standard (11-bit identifier)  MsgIdentifier=644  MsgLength=8  SignalInfo=AC_Max_Power$52$4$2$2$1$0$1$0$0$15$#CompCur_MEAS_Comp$16$8$2$2$1$0$1.250000e-01$0$0$3.187000e+01$#CompSpd_MEAS_Comp$32$16$2$2$1$0$2.500000e-01$0$0$1.638375e+04$#CompVol_MEAS_Comp$8$16$2$2$1$0$1.000000e-01$0$0$6.553400e+03$#InternalVol_ERR_Comp$44$1$2$2$1$0$1$0$0$1$#OverCur_ERR_Comp$41$1$2$2$1$0$1$0$0$1$#OverVol_ERR_Comp$42$1$2$2$1$0$1$0$0$1$#Temp_ERR_Comp$40$1$2$2$1$0$1$0$0$1$#UnderVol_ERR_Comp$43$1$2$2$1$0$1$0$0$1$#Work_STS_Comp$46$2$2$2$1$0$1$0$0$3$#  NSignals=10  IDPort=off  TimestampPort=off  ErrorPort=off  RemotePort=off  LengthPort=off  StatusPort=off  StartBits=str2num('[int32(52);int32(16);int32(32);int32(8);int32(44);int32(41);int32(42);int32(40);int32(43);int32(46)]')  SignalSizes=str2num('[int32(4);int32(8);int32(16);int32(16);int32(1);int32(1);int32(1);int32(1);int32(1);int32(2)]')  ByteOrders=str2num('[int32(2);int32(2);int32(2);int32(2);int32(2);int32(2);int32(2);int32(2);int32(2);int32(2)]')  DataTypes=str2num('[int32(2);int32(2);int32(2);int32(2);int32(2);int32(2);int32(2);int32(2);int32(2);int32(2)]')  MultiplexTypes=str2num('[int32(1);int32(1);int32(1);int32(1);int32(1);int32(1);int32(1);int32(1);int32(1);int32(1)]')  MultiplexValues=str2num('[double(0);double(0);double(0);double(0);double(0);double(0);double(0);double(0);double(0);double(0)]')  Factors=str2num('[double(1);double(1.250000e-01);double(2.500000e-01);double(1.000000e-01);double(1);double(1);double(1);double(1);double(1);double(1)]')  Offsets=str2num('[double(0);double(0);double(0);double(0);double(0);double(0);double(0);double(0);double(0);double(0)]')  Minimums=str2num('[double(0);double(0);double(0);double(0);double(0);double(0);double(0);double(0);double(0);double(0)]')  Maximums=str2num('[double(15);double(3.187000e+01);double(1.638375e+04);double(6.553400e+03);double(1);double(1);double(1);double(1);double(1);double(3)]')  ApplyMinMax=off
      settings: SourceProductName=Simulink Real-Time  SourceProductBaseCode=XP  DataFormat=CANdb specified signals
  Constant : Constant  OutDataTypeStr=uint8
  Constant1 : Constant  Value=0  OutDataTypeStr=uint8
  Constant4 : Constant  Value=0  OutDataTypeStr=uint8
  Constant5 : Constant  Value=0  OutDataTypeStr=uint8
  Data Store Read : DataStoreRead  DataStoreName=Cnt_ACM
  Data Store Write : DataStoreWrite  DataStoreName=Cnt_ACM
  Data Type Conversion{,3,6..10,14..15,17} (10 alike) : DataTypeConversion  OutDataTypeStr=uint8
  Data Type Conversion{1..2,4..5} (4 alike) : DataTypeConversion  OutDataTypeStr=single
  Data Type Conversion18 : DataTypeConversion  OutDataTypeStr=uint32
  Data Type Conversion19 : DataTypeConversion  OutDataTypeStr=double
  Message : Outport
  wires:
  Constant4/1 -> Data Type Conversion15/1
  length/1 -> Data Type Conversion14/1
  data/1 -> Bus Creator/7  "Data"
  Data Type Conversion18/1 -> Bus Creator/5  "ID"
  Constant1/1 -> Data Type Conversion/1
  Constant5/1 -> Data Type Conversion17/1
  ID/1 -> Data Type Conversion18/1
  Data Type Conversion19/1 -> Bus Creator/6  "Timestamp"
  timestamp/1 -> Data Type Conversion19/1
  Data Type Conversion17/1 -> Bus Creator/4  "Error"
  Bus Creator/1 -> CAN Unpack6/1  "CAN_Msg_In"
  Data Type Conversion/1 -> Bus Creator/1  "Extended"
  Data Type Conversion14/1 -> Bus Creator/2  "Length"
  Data Type Conversion15/1 -> Bus Creator/3  "Remote"
  Bus Creator1/1 -> Message/1
  CAN Unpack6/1 -> Data Type Conversion1/1
  CAN Unpack6/2 -> Data Type Conversion4/1
  CAN Unpack6/3 -> Data Type Conversion2/1
  CAN Unpack6/4 -> Data Type Conversion5/1
  CAN Unpack6/5 -> Data Type Conversion3/1
  CAN Unpack6/6 -> Data Type Conversion6/1
  CAN Unpack6/7 -> Data Type Conversion7/1
  CAN Unpack6/8 -> Data Type Conversion8/1
  CAN Unpack6/9 -> Data Type Conversion9/1
  CAN Unpack6/10 -> Data Type Conversion10/1
  Data Type Conversion1/1 -> Bus Creator1/1  "AC_Max_Power"
  Data Type Conversion2/1 -> Bus Creator1/3  "CompSpd_MEAS_Comp"
  Data Type Conversion4/1 -> Bus Creator1/2  "CompCur_MEAS_Comp"
  Data Type Conversion5/1 -> Bus Creator1/4  "CompVol_MEAS_Comp"
  Data Type Conversion3/1 -> Bus Creator1/5  "InternalVol_ERR_Comp"
  Data Type Conversion6/1 -> Bus Creator1/6  "OverCur_ERR_Comp"
  Data Type Conversion7/1 -> Bus Creator1/7  "OverVol_ERR_Comp"
  Data Type Conversion8/1 -> Bus Creator1/8  "Temp_ERR_Comp"
  Data Type Conversion9/1 -> Bus Creator1/9  "UnderVol_ERR_Comp"
  Data Type Conversion10/1 -> Bus Creator1/10  "Work_STS_Comp"
  Constant/1 -> Add/2
  Data Store Read/1 -> Add/1
  Add/1 -> Data Store Write/1

== system VehCtrl20260630_18B/SigIn/CAN1/AVCU_Msg/UNPACK ==
  ID : Inport
  data : Inport  Port=2
  length : Inport  Port=3
  timestamp : Inport  Port=4
  Action Port : ActionPort  ActionType=case
  Add : Sum
  Bus Creator : BusCreator  Inputs=7  OutDataTypeStr=Bus: CAN_MESSAGE_BUS  NonVirtualBus=on
  Bus Creator1 : BusCreator  Inputs=7
  CAN Unpack6 : canmsglib/CAN Unpack  CANdbFile=D:\VCU\VCU_AgriculturalMachinery_ChangChun\CAN协议8.4\液压\BDX_DBC_VCU_CAN0.dbc  MsgList=AVCU_180  MsgName=AVCU_180  MsgIDType=Standard (11-bit identifier)  MsgIdentifier=384  MsgLength=8  SignalInfo=AP_fault$49$1$1$2$1$0$1$0$0$1$#AccumulatorPressure$0$16$1$2$1$0$1$0$0$200$#BP_fault$50$1$1$2$1$0$1$0$0$1$#BrakePressure$16$16$1$2$1$0$1$0$0$200$#PressureSwitch$48$1$1$2$1$0$1$0$0$1$#SA_fault$51$1$1$2$1$0$1$0$0$1$#SteeringAngle$32$16$1$2$1$0$1.000000e-01$-180$-180$6.373500e+03$#  NSignals=7  IDPort=off  TimestampPort=off  ErrorPort=off  RemotePort=off  LengthPort=off  StatusPort=off  StartBits=str2num('[int32(49);int32(0);int32(50);int32(16);int32(48);int32(51);int32(32)]')  SignalSizes=str2num('[int32(1);int32(16);int32(1);int32(16);int32(1);int32(1);int32(16)]')  ByteOrders=str2num('[int32(1);int32(1);int32(1);int32(1);int32(1);int32(1);int32(1)]')  DataTypes=str2num('[int32(2);int32(2);int32(2);int32(2);int32(2);int32(2);int32(2)]')  MultiplexTypes=str2num('[int32(1);int32(1);int32(1);int32(1);int32(1);int32(1);int32(1)]')  MultiplexValues=str2num('[double(0);double(0);double(0);double(0);double(0);double(0);double(0)]')  Factors=str2num('[double(1);double(1);double(1);double(1);double(1);double(1);double(1.000000e-01)]')  Offsets=str2num('[double(0);double(0);double(0);double(0);double(0);double(0);double(-180)]')  Minimums=str2num('[double(0);double(0);double(0);double(0);double(0);double(0);double(-180)]')  Maximums=str2num('[double(1);double(200);double(1);double(200);double(1);double(1);double(6.373500e+03)]')  ApplyMinMax=off
      settings: SourceProductName=Simulink Real-Time  SourceProductBaseCode=XP  DataFormat=CANdb specified signals
  Constant : Constant  OutDataTypeStr=uint8
  Constant1 : Constant  Value=0  OutDataTypeStr=uint8
  Constant4 : Constant  Value=0  OutDataTypeStr=uint8
  Constant5 : Constant  Value=0  OutDataTypeStr=uint8
  Data Store Read : DataStoreRead  DataStoreName=Cnt_BDX
  Data Store Write : DataStoreWrite  DataStoreName=Cnt_BDX
  Data Store Write2 : DataStoreWrite  DataStoreName=SteerAngFR
  Data Type Conversion{,1..4,14..15,17} (8 alike) : DataTypeConversion  OutDataTypeStr=uint8
  Data Type Conversion18 : DataTypeConversion  OutDataTypeStr=uint32
  Data Type Conversion19 : DataTypeConversion  OutDataTypeStr=double
  Data Type Conversion60 : DataTypeConversion  OutDataTypeStr=single
  Data Type Conversion61 : DataTypeConversion  OutDataTypeStr=single
  Data Type Conversion62 : DataTypeConversion  OutDataTypeStr=single
  Message : Outport
  wires:
  Data Type Conversion62/1 -> Data Store Write2/1, Bus Creator1/3  "BDX_SteeringAngle"
  Data Type Conversion61/1 -> Bus Creator1/2  "BDX_BrakePressure"
  Data Type Conversion60/1 -> Bus Creator1/1  "BDX_AccumulatorPressure"
  Bus Creator1/1 -> Message/1
  Data Type Conversion15/1 -> Bus Creator/3  "Remote"
  Data Type Conversion14/1 -> Bus Creator/2  "Length"
  Data Type Conversion/1 -> Bus Creator/1  "Extended"
  Bus Creator/1 -> CAN Unpack6/1  "CAN_Msg_In"
  Data Type Conversion17/1 -> Bus Creator/4  "Error"
  timestamp/1 -> Data Type Conversion19/1
  Data Type Conversion19/1 -> Bus Creator/6  "Timestamp"
  ID/1 -> Data Type Conversion18/1
  Constant5/1 -> Data Type Conversion17/1
  Constant1/1 -> Data Type Conversion/1
  Data Type Conversion18/1 -> Bus Creator/5  "ID"
  data/1 -> Bus Creator/7  "Data"
  length/1 -> Data Type Conversion14/1
  Constant4/1 -> Data Type Conversion15/1
  Data Type Conversion3/1 -> Bus Creator1/7  "BDX_SA_fault"
  CAN Unpack6/2 -> Data Type Conversion60/1
  CAN Unpack6/4 -> Data Type Conversion61/1
  CAN Unpack6/7 -> Data Type Conversion62/1
  CAN Unpack6/6 -> Data Type Conversion3/1
  CAN Unpack6/3 -> Data Type Conversion4/1
  CAN Unpack6/1 -> Data Type Conversion1/1
  CAN Unpack6/5 -> Data Type Conversion2/1
  Data Type Conversion2/1 -> Bus Creator1/4  "BDX_PressureSwitch"
  Data Type Conversion1/1 -> Bus Creator1/5  "BDX_AP_fault"
  Data Type Conversion4/1 -> Bus Creator1/6  "BDX_BP_fault"
  Add/1 -> Data Store Write/1
  Constant/1 -> Add/2
  Data Store Read/1 -> Add/1

== system VehCtrl20260630_18B/SigIn/CAN1/BMS_CANWakeUpID/UNPACK ==
  ID : Inport
  data : Inport  Port=2
  length : Inport  Port=3
  timestamp : Inport  Port=4
  Action Port : ActionPort  ActionType=case
  Bus Creator : BusCreator  Inputs=7  OutDataTypeStr=Bus: CAN_MESSAGE_BUS  NonVirtualBus=on
  Bus Creator1 : BusCreator  Inputs=8
  CAN Unpack6 : canmsglib/CAN Unpack  CANdbFile=D:\VCU\VCU_AgriculturalMachinery_ChangChun\CAN协议8.4\BMS\BMS_DBC_Sheet1.dbc  MsgList=BMS_CANWakeUpID  MsgName=BMS_CANWakeUpID  MsgIDType=Extended (29-bit identifier)  MsgIdentifier=403515719  MsgLength=8  SignalInfo=DB0$0$8$2$2$1$0$1$0$0$255$#DB1$8$8$2$2$1$0$1$0$0$255$#DB2$16$8$2$2$1$0$1$0$0$255$#DB3$24$8$2$2$1$0$1$0$0$255$#DB4$32$8$2$2$1$0$1$0$0$255$#DB5$40$8$2$2$1$0$1$0$0$255$#DB6$48$8$2$2$1$0$1$0$0$255$#DB7$56$8$2$2$1$0$1$0$0$255$#  NSignals=8  IDPort=off  TimestampPort=off  ErrorPort=off  RemotePort=off  LengthPort=off  StatusPort=off  StartBits=str2num('[int32(0);int32(8);int32(16);int32(24);int32(32);int32(40);int32(48);int32(56)]')  SignalSizes=str2num('[int32(8);int32(8);int32(8);int32(8);int32(8);int32(8);int32(8);int32(8)]')  ByteOrders=str2num('[int32(2);int32(2);int32(2);int32(2);int32(2);int32(2);int32(2);int32(2)]')  DataTypes=str2num('[int32(2);int32(2);int32(2);int32(2);int32(2);int32(2);int32(2);int32(2)]')  MultiplexTypes=str2num('[int32(1);int32(1);int32(1);int32(1);int32(1);int32(1);int32(1);int32(1)]')  MultiplexValues=str2num('[double(0);double(0);double(0);double(0);double(0);double(0);double(0);double(0)]')  Factors=str2num('[double(1);double(1);double(1);double(1);double(1);double(1);double(1);double(1)]')  Offsets=str2num('[double(0);double(0);double(0);double(0);double(0);double(0);double(0);double(0)]')  Minimums=str2num('[double(0);double(0);double(0);double(0);double(0);double(0);double(0);double(0)]')  Maximums=str2num('[double(255);double(255);double(255);double(255);double(255);double(255);double(255);double(255)]')  ApplyMinMax=off
      settings: SourceProductName=Simulink Real-Time  SourceProductBaseCode=XP  DataFormat=CANdb specified signals
  Constant1 : Constant  OutDataTypeStr=uint8
  Constant4 : Constant  Value=0  OutDataTypeStr=uint8
  Constant5 : Constant  Value=0  OutDataTypeStr=uint8
  Data Type Conversion{,1..6,9,14..15,17,60} (12 alike) : DataTypeConversion  OutDataTypeStr=uint8
  Data Type Conversion18 : DataTypeConversion  OutDataTypeStr=uint32
  Data Type Conversion19 : DataTypeConversion  OutDataTypeStr=double
  Message : Outport
  wires:
  Bus Creator1/1 -> Message/1
  Data Type Conversion15/1 -> Bus Creator/3  "Remote"
  Data Type Conversion14/1 -> Bus Creator/2  "Length"
  Data Type Conversion/1 -> Bus Creator/1  "Extended"
  Bus Creator/1 -> CAN Unpack6/1  "CAN_Msg_In"
  Data Type Conversion17/1 -> Bus Creator/4  "Error"
  timestamp/1 -> Data Type Conversion19/1
  Data Type Conversion19/1 -> Bus Creator/6  "Timestamp"
  ID/1 -> Data Type Conversion18/1
  Constant5/1 -> Data Type Conversion17/1
  Constant1/1 -> Data Type Conversion/1
  Data Type Conversion18/1 -> Bus Creator/5  "ID"
  data/1 -> Bus Creator/7  "Data"
  length/1 -> Data Type Conversion14/1
  Constant4/1 -> Data Type Conversion15/1
  CAN Unpack6/1 -> Data Type Conversion60/1
  CAN Unpack6/2 -> Data Type Conversion1/1
  CAN Unpack6/3 -> Data Type Conversion2/1
  CAN Unpack6/4 -> Data Type Conversion3/1
  CAN Unpack6/5 -> Data Type Conversion4/1
  CAN Unpack6/6 -> Data Type Conversion9/1
  CAN Unpack6/7 -> Data Type Conversion5/1
  CAN Unpack6/8 -> Data Type Conversion6/1
  Data Type Conversion60/1 -> Bus Creator1/1  "DB0"
  Data Type Conversion1/1 -> Bus Creator1/2  "DB1"
  Data Type Conversion2/1 -> Bus Creator1/3  "DB2"
  Data Type Conversion3/1 -> Bus Creator1/4  "DB3"
  Data Type Conversion4/1 -> Bus Creator1/5  "DB4"
  Data Type Conversion9/1 -> Bus Creator1/6  "DB5"
  Data Type Conversion5/1 -> Bus Creator1/7  "DB6"
  Data Type Conversion6/1 -> Bus Creator1/8  "DB7"

== system VehCtrl20260630_18B/SigIn/CAN1/BMS_CellTempCycTx/UNPACK ==
  ID : Inport
  data : Inport  Port=2
  length : Inport  Port=3
  timestamp : Inport  Port=4
  Action Port : ActionPort  ActionType=case
  Bus Creator : BusCreator  Inputs=7  OutDataTypeStr=Bus: CAN_MESSAGE_BUS  NonVirtualBus=on
  Bus Creator1 : BusCreator  Inputs=8
  CAN Unpack6 : canmsglib/CAN Unpack  CANdbFile=D:\VCU\VCU_AgriculturalMachinery_ChangChun\CAN协议8.4\BMS\BMS_DBC_Sheet1.dbc  MsgList=BMS_CellTempCycTx  MsgName=BMS_CellTempCycTx  MsgIDType=Extended (29-bit identifier)  MsgIdentifier=408955207  MsgLength=8  SignalInfo=BMS_CellTempGroupNum$0$8$2$2$1$0$1$0$1$255$#BMS_CellTemp_n0$8$8$2$2$1$0$1$-40$-40$125$#BMS_CellTemp_n1$16$8$2$2$1$0$1$-40$-40$125$#BMS_CellTemp_n2$24$8$2$2$1$0$1$-40$-40$125$#BMS_CellTemp_n3$32$8$2$2$1$0$1$-40$-40$125$#BMS_CellTemp_n4$40$8$2$2$1$0$1$-40$-40$125$#BMS_CellTemp_n5$48$8$2$2$1$0$1$-40$-40$125$#BMS_CellTemp_n6$56$8$2$2$1$0$1$-40$-40$125$#  NSignals=8  IDPort=off  TimestampPort=off  ErrorPort=off  RemotePort=off  LengthPort=off  StatusPort=off  StartBits=str2num('[int32(0);int32(8);int32(16);int32(24);int32(32);int32(40);int32(48);int32(56)]')  SignalSizes=str2num('[int32(8);int32(8);int32(8);int32(8);int32(8);int32(8);int32(8);int32(8)]')  ByteOrders=str2num('[int32(2);int32(2);int32(2);int32(2);int32(2);int32(2);int32(2);int32(2)]')  DataTypes=str2num('[int32(2);int32(2);int32(2);int32(2);int32(2);int32(2);int32(2);int32(2)]')  MultiplexTypes=str2num('[int32(1);int32(1);int32(1);int32(1);int32(1);int32(1);int32(1);int32(1)]')  MultiplexValues=str2num('[double(0);double(0);double(0);double(0);double(0);double(0);double(0);double(0)]')  Factors=str2num('[double(1);double(1);double(1);double(1);double(1);double(1);double(1);double(1)]')  Offsets=str2num('[double(0);double(-40);double(-40);double(-40);double(-40);double(-40);double(-40);double(-40)]')  Minimums=str2num('[double(1);double(-40);double(-40);double(-40);double(-40);double(-40);double(-40);double(-40)]')  Maximums=str2num('[double(255);double(125);double(125);double(125);double(125);double(125);double(125);double(125)]')  ApplyMinMax=off
      settings: SourceProductName=Simulink Real-Time  SourceProductBaseCode=XP  DataFormat=CANdb specified signals
  Constant1 : Constant  OutDataTypeStr=uint8
  Constant4 : Constant  Value=0  OutDataTypeStr=uint8
  Constant5 : Constant  Value=0  OutDataTypeStr=uint8
  Data Type Conversion{,14..15,17} (4 alike) : DataTypeConversion  OutDataTypeStr=uint8
  Data Type Conversion{1..6,9,60} (8 alike) : DataTypeConversion  OutDataTypeStr=single
  Data Type Conversion18 : DataTypeConversion  OutDataTypeStr=uint32
  Data Type Conversion19 : DataTypeConversion  OutDataTypeStr=double
  Message : Outport
  wires:
  Bus Creator1/1 -> Message/1
  Data Type Conversion15/1 -> Bus Creator/3  "Remote"
  Data Type Conversion14/1 -> Bus Creator/2  "Length"
  Data Type Conversion/1 -> Bus Creator/1  "Extended"
  Bus Creator/1 -> CAN Unpack6/1  "CAN_Msg_In"
  Data Type Conversion17/1 -> Bus Creator/4  "Error"
  timestamp/1 -> Data Type Conversion19/1
  Data Type Conversion19/1 -> Bus Creator/6  "Timestamp"
  ID/1 -> Data Type Conversion18/1
  Constant5/1 -> Data Type Conversion17/1
  Constant1/1 -> Data Type Conversion/1
  Data Type Conversion18/1 -> Bus Creator/5  "ID"
  data/1 -> Bus Creator/7  "Data"
  length/1 -> Data Type Conversion14/1
  Constant4/1 -> Data Type Conversion15/1
  Data Type Conversion5/1 -> Bus Creator1/7  "BMS_CellTemp_n5"
  Data Type Conversion6/1 -> Bus Creator1/8  "BMS_CellTemp_n6"
  Data Type Conversion3/1 -> Bus Creator1/4  "BMS_CellTemp_n2"
  Data Type Conversion2/1 -> Bus Creator1/3  "BMS_CellTemp_n1"
  Data Type Conversion4/1 -> Bus Creator1/5  "BMS_CellTemp_n3"
  Data Type Conversion1/1 -> Bus Creator1/2  "BMS_CellTemp_n0"
  Data Type Conversion9/1 -> Bus Creator1/6  "BMS_CellTemp_n4"
  Data Type Conversion60/1 -> Bus Creator1/1  "BMS_CellTempGroupNum"
  CAN Unpack6/1 -> Data Type Conversion60/1
  CAN Unpack6/2 -> Data Type Conversion1/1
  CAN Unpack6/3 -> Data Type Conversion2/1
  CAN Unpack6/4 -> Data Type Conversion3/1
  CAN Unpack6/5 -> Data Type Conversion4/1
  CAN Unpack6/6 -> Data Type Conversion9/1
  CAN Unpack6/7 -> Data Type Conversion5/1
  CAN Unpack6/8 -> Data Type Conversion6/1
